simulink model "rlKinovaBallBalance"  (R2024a)
settings: Solver=ode15s  StartTime=0.0  StopTime=10  RelTol=1e-3  AbsTol=1e-3
undefined symbols (not defined in the file or in its folder): ball, g, max_torque, plate, R1_q0, R2_q0, R3_q0, R4_q0, R5_q0, U0, X, Y, Z
libraries: sm_lib x96, nesl_utility_internal x18, simulink x2, rllib x1
(part 3 of 3)

== system rlKinovaBallBalance/Kinova Ball Balance/7 DOF Manipulator/Bracelet_Link/Bracelet Link/Inertia ==
  Inertia1 : sm_lib/Body Elements/Inertia  InertiaType=Custom  Mass=0.0639903  MassUnits=kg  CenterOfMass=[-0.000374733, 0.0200972, 0.0397002]  CenterOfMassUnits=m  MomentsOfInertia=[8.77763e-05, 5.386e-05, 0.000111032]  MomentsOfInertiaUnits=kg*m^2  ProductsOfInertia=[-7.81917e-06, 1.77829e-07, -4.01652e-07]  ProductsOfInertiaUnits=kg*m^2  GraphicType=Marker  MarkerShape=Inertia  MarkerSize=20  GraphicVisPropType=SimpleVisualProperties  GraphicDiffuseColor=[0.5 0.5 0.5]  GraphicOpacity=1.0  GraphicSpecularColor=[0.5 0.5 0.5 1.0]  GraphicAmbientColor=[0.15 0.15 0.15 1.0]  GraphicEmissiveColor=[0.0 0.0 0.0 1.0]  GraphicShininess=75
  R : PMIOPort  Side=Right
  connections:
  Inertia1/RConn1 -- R/RConn1

== system rlKinovaBallBalance/Kinova Ball Balance/7 DOF Manipulator/ForeArm_Link/ForeArm Link/FileSolid ==
  Forearm Link : sm_lib/Body Elements/File Solid  ExtGeomFileName=forearm_link.STL  UnitType=Custom  ExtGeomFileUnits=m  StepReaderType=HEX  ExportConvexHullGeometry=off  InertiaType=Custom  Mass=0.108759  MassUnits=kg  CenterOfMass=[0.0794976, 0.0148416, -8.39544e-07]  CenterOfMassUnits=m  MomentsOfInertia=[0.000118324, 0.000832188, 0.000809477]  MomentsOfInertiaUnits=kg*m^2  ProductsOfInertia=[3.60538e-09, -2.24072e-09, 7.50733e-05]  ProductsOfInertiaUnits=kg*m^2  BasedOnType=DensityFromFile  Density=1000  DensityUnits=kg/m^3  DoExposeReferenceFrame=on  SerializedFrames=<Frames/>  GraphicType=FromGeometry  MarkerShape=Sphere  MarkerSize=10  GraphicVisPropType=SimpleVisualProperties  GraphicDiffuseColor=[0.54509807 0.654902 0.77254903]  GraphicSpecularColor=[0.5 0.5 0.5 1.0]  GraphicAmbientColor=[0.15 0.15 0.15 1.0]  GraphicEmissiveColor=[0.0 0.0 0.0 1.0]  GraphicShininess=75  GraphicOpacity=1
  R : PMIOPort  Side=Right
  connections:
  Forearm Link/RConn1 -- R/RConn1

== system rlKinovaBallBalance/Kinova Ball Balance/7 DOF Manipulator/ForeArm_Link/ForeArm Link/Inertia ==
  Inertia1 : sm_lib/Body Elements/Inertia  InertiaType=Custom  Mass=0.108759  MassUnits=kg  CenterOfMass=[0.0794976, 0.0148416, -8.39544e-07]  CenterOfMassUnits=m  MomentsOfInertia=[0.000118324, 0.000832188, 0.000809477]  MomentsOfInertiaUnits=kg*m^2  ProductsOfInertia=[3.60538e-09, -2.24072e-09, 7.50733e-05]  ProductsOfInertiaUnits=kg*m^2  GraphicType=Marker  MarkerShape=Inertia  MarkerSize=20  GraphicVisPropType=SimpleVisualProperties  GraphicDiffuseColor=[0.5 0.5 0.5]  GraphicOpacity=1.0  GraphicSpecularColor=[0.5 0.5 0.5 1.0]  GraphicAmbientColor=[0.15 0.15 0.15 1.0]  GraphicEmissiveColor=[0.0 0.0 0.0 1.0]  GraphicShininess=75
  R : PMIOPort  Side=Right
  connections:
  Inertia1/RConn1 -- R/RConn1

== system rlKinovaBallBalance/Kinova Ball Balance/7 DOF Manipulator/HalfArm1_Link/HalfArm1 Link/FileSolid ==
  Half Arm1 Link : sm_lib/Body Elements/File Solid  ExtGeomFileName=half_arm_1_link.STL  UnitType=Custom  ExtGeomFileUnits=m  StepReaderType=HEX  ExportConvexHullGeometry=off  InertiaType=Custom  Mass=0.137977  MassUnits=kg  CenterOfMass=[0.100808, 0.0121234, 4.10274e-06]  CenterOfMassUnits=m  MomentsOfInertia=[0.000202425, 0.00113112, 0.00110619]  MomentsOfInertiaUnits=kg*m^2  ProductsOfInertia=[1.72409e-08, -8.98835e-09, 0.000105223]  ProductsOfInertiaUnits=kg*m^2  BasedOnType=DensityFromFile  Density=1000  DensityUnits=kg/m^3  DoExposeReferenceFrame=on  SerializedFrames=<Frames/>  GraphicType=FromGeometry  MarkerShape=Sphere  MarkerSize=10  GraphicVisPropType=SimpleVisualProperties  GraphicDiffuseColor=[0.54509807 0.654902 0.77254903]  GraphicSpecularColor=[0.5 0.5 0.5 1.0]  GraphicAmbientColor=[0.15 0.15 0.15 1.0]  GraphicEmissiveColor=[0.0 0.0 0.0 1.0]  GraphicShininess=75  GraphicOpacity=1
  R : PMIOPort  Side=Right
  connections:
  Half Arm1 Link/RConn1 -- R/RConn1

== system rlKinovaBallBalance/Kinova Ball Balance/7 DOF Manipulator/HalfArm1_Link/HalfArm1 Link/Inertia ==
  Inertia1 : sm_lib/Body Elements/Inertia  InertiaType=Custom  Mass=0.137977  MassUnits=kg  CenterOfMass=[0.100808, 0.0121234, 4.10274e-06]  CenterOfMassUnits=m  MomentsOfInertia=[0.000202425, 0.00113112, 0.00110619]  MomentsOfInertiaUnits=kg*m^2  ProductsOfInertia=[1.72409e-08, -8.98835e-09, 0.000105223]  ProductsOfInertiaUnits=kg*m^2  GraphicType=Marker  MarkerShape=Inertia  MarkerSize=20  GraphicVisPropType=SimpleVisualProperties  GraphicDiffuseColor=[0.5 0.5 0.5]  GraphicOpacity=1.0  GraphicSpecularColor=[0.5 0.5 0.5 1.0]  GraphicAmbientColor=[0.15 0.15 0.15 1.0]  GraphicEmissiveColor=[0.0 0.0 0.0 1.0]  GraphicShininess=75
  R : PMIOPort  Side=Right
  connections:
  Inertia1/RConn1 -- R/RConn1

== system rlKinovaBallBalance/Kinova Ball Balance/7 DOF Manipulator/HalfArm2_Link/HalfArm2 Link/FileSolid ==
  Half Arm2 Link : sm_lib/Body Elements/File Solid  ExtGeomFileName=half_arm_2_link.STL  UnitType=Custom  ExtGeomFileUnits=m  StepReaderType=HEX  ExportConvexHullGeometry=off  InertiaType=Custom  Mass=0.137978  MassUnits=kg  CenterOfMass=[0.0871838, 0.0118108, 4.16659e-06]  CenterOfMassUnits=m  MomentsOfInertia=[0.000195075, 0.0011006, 0.00106833]  MomentsOfInertiaUnits=kg*m^2  ProductsOfInertia=[1.66656e-08, -1.69023e-08, 7.86653e-05]  ProductsOfInertiaUnits=kg*m^2  BasedOnType=DensityFromFile  Density=1000  DensityUnits=kg/m^3  DoExposeReferenceFrame=on  SerializedFrames=<Frames/>  GraphicType=FromGeometry  MarkerShape=Sphere  MarkerSize=10  GraphicVisPropType=SimpleVisualProperties  GraphicDiffuseColor=[0.6666667 0.77254903 0.92941177]  GraphicSpecularColor=[0.5 0.5 0.5 1.0]  GraphicAmbientColor=[0.15 0.15 0.15 1.0]  GraphicEmissiveColor=[0.0 0.0 0.0 1.0]  GraphicShininess=75  GraphicOpacity=1
  R : PMIOPort  Side=Right
  connections:
  Half Arm2 Link/RConn1 -- R/RConn1

== system rlKinovaBallBalance/Kinova Ball Balance/7 DOF Manipulator/HalfArm2_Link/HalfArm2 Link/Inertia ==
  Inertia1 : sm_lib/Body Elements/Inertia  InertiaType=Custom  Mass=0.137978  MassUnits=kg  CenterOfMass=[0.0871838, 0.0118108, 4.16659e-06]  CenterOfMassUnits=m  MomentsOfInertia=[0.000195075, 0.0011006, 0.00106833]  MomentsOfInertiaUnits=kg*m^2  ProductsOfInertia=[1.66656e-08, -1.69023e-08, 7.86653e-05]  ProductsOfInertiaUnits=kg*m^2  GraphicType=Marker  MarkerShape=Inertia  MarkerSize=20  GraphicVisPropType=SimpleVisualProperties  GraphicDiffuseColor=[0.5 0.5 0.5]  GraphicOpacity=1.0  GraphicSpecularColor=[0.5 0.5 0.5 1.0]  GraphicAmbientColor=[0.15 0.15 0.15 1.0]  GraphicEmissiveColor=[0.0 0.0 0.0 1.0]  GraphicShininess=75
  R : PMIOPort  Side=Right
  connections:
  Inertia1/RConn1 -- R/RConn1

== system rlKinovaBallBalance/Kinova Ball Balance/7 DOF Manipulator/Shoulder_Link/Shoulder Link/FileSolid ==
  Shoulder Link : sm_lib/Body Elements/File Solid  ExtGeomFileName=shoulder_link.STL  UnitType=Custom  ExtGeomFileUnits=m  StepReaderType=HEX  ExportConvexHullGeometry=off  InertiaType=Custom  Mass=0.206679  MassUnits=kg  CenterOfMass=[0.0758362, 0.0170163, 7.48345e-07]  CenterOfMassUnits=m  MomentsOfInertia=[0.000301623, 0.000658228, 0.000584422]  MomentsOfInertiaUnits=kg*m^2  ProductsOfInertia=[6.12368e-09, 4.93274e-09, -6.36892e-05]  ProductsOfInertiaUnits=kg*m^2  BasedOnType=DensityFromFile  Density=1000  DensityUnits=kg/m^3  DoExposeReferenceFrame=on  SerializedFrames=<Frames/>  GraphicType=FromGeometry  MarkerShape=Sphere  MarkerSize=10  GraphicVisPropType=SimpleVisualProperties  GraphicDiffuseColor=[0.6666667 0.77254903 0.92941177]  GraphicSpecularColor=[0.5 0.5 0.5 1.0]  GraphicAmbientColor=[0.15 0.15 0.15 1.0]  GraphicEmissiveColor=[0.0 0.0 0.0 1.0]  GraphicShininess=75  GraphicOpacity=1
  R : PMIOPort  Side=Right
  connections:
  R/RConn1 -- Shoulder Link/RConn1

== system rlKinovaBallBalance/Kinova Ball Balance/7 DOF Manipulator/Shoulder_Link/Shoulder Link/Inertia ==
  Inertia1 : sm_lib/Body Elements/Inertia  InertiaType=Custom  Mass=0.206679  MassUnits=kg  CenterOfMass=[0.0758362, 0.0170163, 7.48345e-07]  CenterOfMassUnits=m  MomentsOfInertia=[0.000301623, 0.000658228, 0.000584422]  MomentsOfInertiaUnits=kg*m^2  ProductsOfInertia=[6.12368e-09, 4.93274e-09, -6.36892e-05]  ProductsOfInertiaUnits=kg*m^2  GraphicType=Marker  MarkerShape=Inertia  MarkerSize=20  GraphicVisPropType=SimpleVisualProperties  GraphicDiffuseColor=[0.5 0.5 0.5]  GraphicOpacity=1.0  GraphicSpecularColor=[0.5 0.5 0.5 1.0]  GraphicAmbientColor=[0.15 0.15 0.15 1.0]  GraphicEmissiveColor=[0.0 0.0 0.0 1.0]  GraphicShininess=75
  R : PMIOPort  Side=Right
  connections:
  Inertia1/RConn1 -- R/RConn1

== system rlKinovaBallBalance/Kinova Ball Balance/7 DOF Manipulator/Wrist1_Link/Wrist1 Link/FileSolid ==
  Wrist1 Link : sm_lib/Body Elements/File Solid  ExtGeomFileName=spherical_wrist_1_link.STL  UnitType=Custom  ExtGeomFileUnits=m  StepReaderType=HEX  ExportConvexHullGeometry=off  InertiaType=Custom  Mass=0.0607261  MassUnits=kg  CenterOfMass=[0.0669267, 0.0134734, -3.64177e-07]  CenterOfMassUnits=m  MomentsOfInertia=[5.88928e-05, 0.000140521, 0.000138155]  MomentsOfInertiaUnits=kg*m^2  ProductsOfInertia=[2.83121e-09, 1.56006e-09, -2.20674e-05]  ProductsOfInertiaUnits=kg*m^2  BasedOnType=DensityFromFile  Density=1000  DensityUnits=kg/m^3  DoExposeReferenceFrame=on  SerializedFrames=<Frames/>  GraphicType=FromGeometry  MarkerShape=Sphere  MarkerSize=10  GraphicVisPropType=SimpleVisualProperties  GraphicDiffuseColor=[0.6666667 0.77254903 0.92941177]  GraphicSpecularColor=[0.5 0.5 0.5 1.0]  GraphicAmbientColor=[0.15 0.15 0.15 1.0]  GraphicEmissiveColor=[0.0 0.0 0.0 1.0]  GraphicShininess=75  GraphicOpacity=1
  R : PMIOPort  Side=Right
  connections:
  Wrist1 Link/RConn1 -- R/RConn1

== system rlKinovaBallBalance/Kinova Ball Balance/7 DOF Manipulator/Wrist1_Link/Wrist1 Link/Inertia ==
  Inertia1 : sm_lib/Body Elements/Inertia  InertiaType=Custom  Mass=0.0607261  MassUnits=kg  CenterOfMass=[0.0669267, 0.0134734, -3.64177e-07]  CenterOfMassUnits=m  MomentsOfInertia=[5.88928e-05, 0.000140521, 0.000138155]  MomentsOfInertiaUnits=kg*m^2  ProductsOfInertia=[2.83121e-09, 1.56006e-09, -2.20674e-05]  ProductsOfInertiaUnits=kg*m^2  GraphicType=Marker  MarkerShape=Inertia  MarkerSize=20  GraphicVisPropType=SimpleVisualProperties  GraphicDiffuseColor=[0.5 0.5 0.5]  GraphicOpacity=1.0  GraphicSpecularColor=[0.5 0.5 0.5 1.0]  GraphicAmbientColor=[0.15 0.15 0.15 1.0]  GraphicEmissiveColor=[0.0 0.0 0.0 1.0]  GraphicShininess=75
  R : PMIOPort  Side=Right
  connections:
  Inertia1/RConn1 -- R/RConn1

== system rlKinovaBallBalance/Kinova Ball Balance/7 DOF Manipulator/Wrist2_Link/Wrist2 Link/FileSolid ==
  Wrist2 Link : sm_lib/Body Elements/File Solid  ExtGeomFileName=spherical_wrist_2_link.STL  UnitType=Custom  ExtGeomFileUnits=m  StepReaderType=HEX  ExportConvexHullGeometry=off  InertiaType=Custom  Mass=0.0607235  MassUnits=kg  CenterOfMass=[0.0566892, 0.0133552, 2.07599e-07]  CenterOfMassUnits=m  MomentsOfInertia=[6.22269e-05, 0.000150545, 0.000151516]  MomentsOfInertiaUnits=kg*m^2  ProductsOfInertia=[-8.5602e-09, -1.23542e-08, -3.01223e-05]  ProductsOfInertiaUnits=kg*m^2  BasedOnType=DensityFromFile  Density=1000  DensityUnits=kg/m^3  DoExposeReferenceFrame=on  SerializedFrames=<Frames/>  GraphicType=FromGeometry  MarkerShape=Sphere  MarkerSize=10  GraphicVisPropType=SimpleVisualProperties  GraphicDiffuseColor=[0.54509807 0.654902 0.77254903]  GraphicSpecularColor=[0.5 0.5 0.5 1.0]  GraphicAmbientColor=[0.15 0.15 0.15 1.0]  GraphicEmissiveColor=[0.0 0.0 0.0 1.0]  GraphicShininess=75  GraphicOpacity=1
  R : PMIOPort  Side=Right
  connections:
  Wrist2 Link/RConn1 -- R/RConn1

== system rlKinovaBallBalance/Kinova Ball Balance/7 DOF Manipulator/Wrist2_Link/Wrist2 Link/Inertia ==
  Inertia1 : sm_lib/Body Elements/Inertia  InertiaType=Custom  Mass=0.0607235  MassUnits=kg  CenterOfMass=[0.0566892, 0.0133552, 2.07599e-07]  CenterOfMassUnits=m  MomentsOfInertia=[6.22269e-05, 0.000150545, 0.000151516]  MomentsOfInertiaUnits=kg*m^2  ProductsOfInertia=[-8.5602e-09, -1.23542e-08, -3.01223e-05]  ProductsOfInertiaUnits=kg*m^2  GraphicType=Marker  MarkerShape=Inertia  MarkerSize=20  GraphicVisPropType=SimpleVisualProperties  GraphicDiffuseColor=[0.5 0.5 0.5]  GraphicOpacity=1.0  GraphicSpecularColor=[0.5 0.5 0.5 1.0]  GraphicAmbientColor=[0.15 0.15 0.15 1.0]  GraphicEmissiveColor=[0.0 0.0 0.0 1.0]  GraphicShininess=75
  R : PMIOPort  Side=Right
  connections:
  Inertia1/RConn1 -- R/RConn1

== system rlKinovaBallBalance/Kinova Ball Balance/7 DOF Manipulator/base_link/Base Link/FileSolid ==
  Base Link : sm_lib/Body Elements/File Solid  ExtGeomFileName=base_link.STL  UnitType=Custom  ExtGeomFileUnits=m  StepReaderType=HEX  ExportConvexHullGeometry=off  InertiaType=Custom  Mass=1.06185  MassUnits=kg  CenterOfMass=[0.000712614, 0.0763467, 0.000106583]  CenterOfMassUnits=m  MomentsOfInertia=[0.00275492, 0.0011525, 0.00277912]  MomentsOfInertiaUnits=kg*m^2  ProductsOfInertia=[-1.84082e-06, 1.0557e-07, 2.81404e-05]  ProductsOfInertiaUnits=kg*m^2  BasedOnType=DensityFromFile  Density=1000  DensityUnits=kg/m^3  DoExposeReferenceFrame=on  SerializedFrames=<Frames/>  GraphicType=FromGeometry  MarkerShape=Sphere  MarkerSize=10  GraphicVisPropType=SimpleVisualProperties  GraphicDiffuseColor=[0.54509807 0.654902 0.77254903]  GraphicSpecularColor=[0.5 0.5 0.5 1.0]  GraphicAmbientColor=[0.15 0.15 0.15 1.0]  GraphicEmissiveColor=[0.0 0.0 0.0 1.0]  GraphicShininess=75  GraphicOpacity=1
  R : PMIOPort  Side=Right
  connections:
  Base Link/RConn1 -- R/RConn1

== system rlKinovaBallBalance/Kinova Ball Balance/7 DOF Manipulator/base_link/Base Link/Inertia ==
  Inertia : sm_lib/Body Elements/Inertia  InertiaType=Custom  Mass=1.06185  MassUnits=kg  CenterOfMass=[0.000712614, 0.0763467, 0.000106583]  CenterOfMassUnits=m  MomentsOfInertia=[0.00275492, 0.0011525, 0.00277912]  MomentsOfInertiaUnits=kg*m^2  ProductsOfInertia=[-1.84082e-06, 1.0557e-07, 2.81404e-05]  ProductsOfInertiaUnits=kg*m^2  GraphicType=Marker  MarkerShape=Inertia  MarkerSize=20  GraphicVisPropType=SimpleVisualProperties  GraphicDiffuseColor=[0.5 0.5 0.5]  GraphicOpacity=1.0  GraphicSpecularColor=[0.5 0.5 0.5 1.0]  GraphicAmbientColor=[0.15 0.15 0.15 1.0]  GraphicEmissiveColor=[0.0 0.0 0.0 1.0]  GraphicShininess=75
  R : PMIOPort  Side=Right
  connections:
  Inertia/RConn1 -- R/RConn1

== matlab function rlKinovaBallBalance/Kinova Ball Balance/Reward/Quaternions to Rotation Angles ZYX sequence ==
  data: q input; tilt output
function tilt = quat2tilt(q)
% Quaternion to Euler angle transformation
% Source: https://en.wikipedia.org/wiki/Conversion_between_quaternions_and_Euler_angles

% unpack quaternion
q0 = q(1);
q1 = q(2);
q2 = q(3);
q3 = q(4);

tilt = zeros(3,1);

% tilt about X axis (tilt_y or roll)
tilt(3) = atan2(2*(q0*q1+q2*q3),1-2*(q1^2+q2^2));

% tilt about Y axis (tilt_x or pitch)
tilt(2) = asin(2*(q0*q2-q3*q1));

% tilt about Z axis (yaw)
tilt(1) = 0;
